simulink model "p9_Sim_State_Space_Diagram"  (R2017b)
settings: Solver=ode14x  StartTime=0.0  StopTime=3  FixedStep=.001  RelTol=1e-3
settings Model: Creator=Harrison  LastModifiedBy=Harrison
settings DataIOCC: SaveFormat=Array

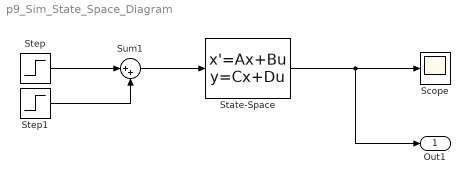
== system p9_Sim_State_Space_Diagram ==
  Scope : Scope
  State-Space : StateSpace  A=[0 1; -3*100/.8 -12*.5/.8/.6^2]  B=[0; 6/.8/.6]  C=[1 0]  D=[0]  InitialCondition=0
  Step : Step  Time=0  After=10  SampleTime=0
  Step1 : Step  Time=.1  After=-10  SampleTime=0
  Sum1 : Sum  Inputs=|++
  Out1 : Outport
  wires:
  Step/1 -> Sum1/1
  Step1/1 -> Sum1/2
  Sum1/1 -> State-Space/1
  State-Space/1 -> Out1/1, Scope/1
